simulink model "MA_simula_dsrac"  (R2012b)
settings: Solver=ode3  StartTime=0  StopTime=Tsim  FixedStep=1e-7  RelTol=1e-3
values from neighbouring files (symbols this model uses):
  D0 = 0.3    [MA_roda_sim.m]    (also in MF_roda_sim_disc.m; sim_padrao.mat = [0.344368016885 0.340474742468 0.337081858539 0.333995318743)
  dD = 0.01    [MA_roda_sim.m]
  dVin = 2    [MA_roda_sim.m]    (also in MF_roda_sim_disc.m)
  tdD = Tsim/3    (= 0.0333333333333)    [MA_roda_sim.m]
  tdVin = 2*Tsim/3    (= 0.0666666666667)    [MA_roda_sim.m]    (also in MF_roda_sim_disc.m = 0.2)
  Vin0 = 15.5    [MA_roda_sim.m]    (also in MF_roda_sim_disc.m)
undefined symbols (not defined in the file or in its folder): A_linear, B_mimo, C, tf_G_den, tf_G_num, tf_Gq_den, tf_Gq_num, xss
settings Model: CovModelRefEnable=off  Creator=jv_flores  LastModifiedBy=anton
settings DataIOCC: LimitDataPoints=off  SaveFormat=StructureWithTime
settings OptimizationCC: ExpressionDepthLimit=128
settings DebuggingCC: UnderspecifiedInitializationDetection=Simplified  MergeDetectMultiDrivingBlocksExec=error  SolverPrmCheckMsg=none  FrameProcessingCompatibilityMsg=error  StateNameClashWarn=none
settings HardwareCC: ProdBitPerPointer=64  ProdLargestAtomicFloat=Float  ProdIntDivRoundTo=Zero  ProdEndianess=LittleEndian  ProdHWDeviceType=Specified
settings ModelReferenceCC: PropagateSignalLabelsOutOfModel=on
settings CodeAppCC: CustomSymbolStrType=$N$R$M_T
settings GRTTargetCC: CodeReplacementLibrary=C89/C90 (ANSI)

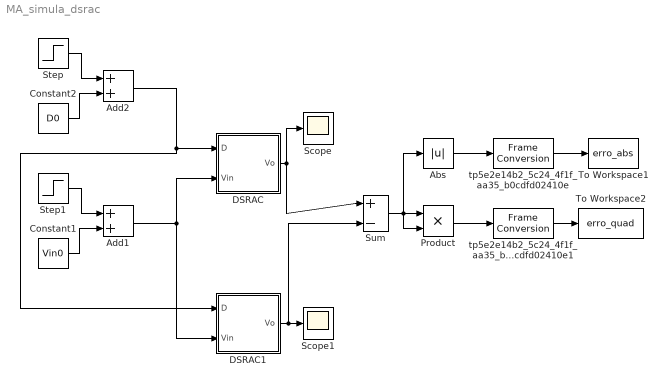
== system MA_simula_dsrac ==
  Abs : Abs
  Add1 : Sum
  Add2 : Sum
  Constant1 : Constant  Value=Vin0
  Constant2 : Constant  Value=D0
  DSRAC : Subsystem
  DSRAC1 : Subsystem
  Product : Product  RndMeth=Zero
  Scope : Scope
      settings: YMin=85.41748  YMax=114.83518
  Scope1 : Scope
      settings: YMin=85.41748  YMax=114.83518
  Step : Step  Time=tdD  After=dD  SampleTime=0
  Step1 : Step  Time=tdVin  After=dVin  SampleTime=0
  Sum : Sum  Inputs=|+-
  To Workspace1 : ToWorkspace  VariableName=erro_abs  SampleTime=-1
  To Workspace2 : ToWorkspace  VariableName=erro_quad  SampleTime=-1
  tp5e2e14b2_5c24_4f1f_aa35_b0cdfd02410e : FrameConversion  OutFrame=Sample-based
  tp5e2e14b2_5c24_4f1f_aa35_b0cdfd02410e1 : FrameConversion  OutFrame=Sample-based
  wires:
  DSRAC/1(Vo) -> Sum/1, Scope/1
  Step/1 -> Add2/1
  Constant2/1 -> Add2/2
  Add2/1 -> DSRAC1/1(D), DSRAC/1(D)
  Step1/1 -> Add1/1
  Constant1/1 -> Add1/2
  Add1/1 -> DSRAC/2(Vin), DSRAC1/2(Vin)
  DSRAC1/1(Vo) -> Sum/2, Scope1/1
  Sum/1 -> Abs/1, Product/2, Product/1
  tp5e2e14b2_5c24_4f1f_aa35_b0cdfd02410e/1 -> To Workspace1/1
  tp5e2e14b2_5c24_4f1f_aa35_b0cdfd02410e1/1 -> To Workspace2/1
  Product/1 -> tp5e2e14b2_5c24_4f1f_aa35_b0cdfd02410e1/1
  Abs/1 -> tp5e2e14b2_5c24_4f1f_aa35_b0cdfd02410e/1

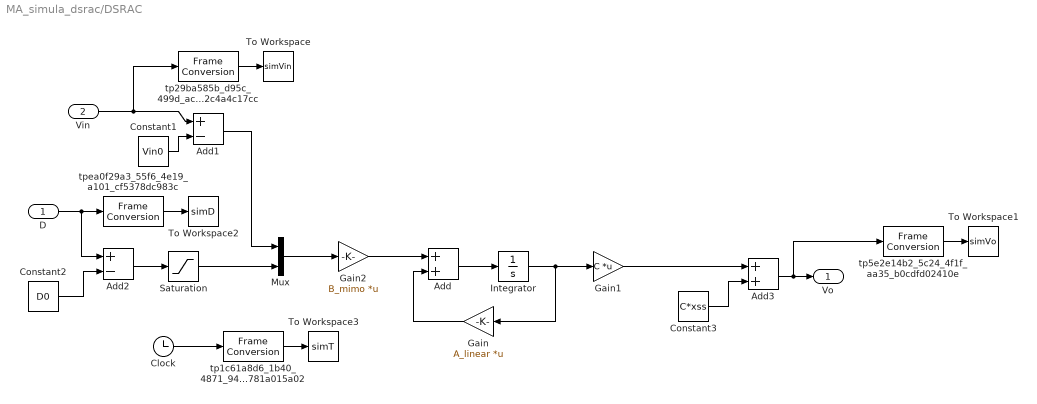
== system MA_simula_dsrac/DSRAC ==
  D : Inport
  Vin : Inport  Port=2
  Add : Sum
  Add1 : Sum  Inputs=+-
  Add2 : Sum  Inputs=+-
  Add3 : Sum
  Clock : Clock
  Constant1 : Constant  Value=Vin0
  Constant2 : Constant  Value=D0
  Constant3 : Constant  Value=C*xss
  Gain : Gain  Gain=A_linear  Multiplication=Matrix(K*u)
  Gain1 : Gain  Gain=C  Multiplication=Matrix(K*u)
  Gain2 : Gain  Gain=B_mimo  Multiplication=Matrix(K*u)
  Integrator : Integrator
  Mux : Mux  Inputs=2
  Saturation : Saturate  UpperLimit=1  LowerLimit=0
  To Workspace : ToWorkspace  VariableName=simVin  SampleTime=-1
  To Workspace1 : ToWorkspace  VariableName=simVo  SampleTime=-1
  To Workspace2 : ToWorkspace  VariableName=simD  SampleTime=-1
  To Workspace3 : ToWorkspace  VariableName=simT  SampleTime=-1
  tp1c61a8d6_1b40_4871_940a_a1781a015a02 : FrameConversion  OutFrame=Sample-based
  tp29ba585b_d95c_499d_aca0_992c4a4c17cc : FrameConversion  OutFrame=Sample-based
  tp5e2e14b2_5c24_4f1f_aa35_b0cdfd02410e : FrameConversion  OutFrame=Sample-based
  tpea0f29a3_55f6_4e19_a101_cf5378dc983c : FrameConversion  OutFrame=Sample-based
  Vo : Outport
  wires:
  Gain2/1 -> Add/1
  Add2/1 -> Saturation/1
  Constant2/1 -> Add2/2
  Integrator/1 -> Gain/1, Gain1/1
  Mux/1 -> Gain2/1
  Gain/1 -> Add/2
  Add/1 -> Integrator/1
  Add3/1 -> Vo/1, tp5e2e14b2_5c24_4f1f_aa35_b0cdfd02410e/1
  Gain1/1 -> Add3/1
  Constant3/1 -> Add3/2
  D/1 -> Add2/1, tpea0f29a3_55f6_4e19_a101_cf5378dc983c/1
  Saturation/1 -> Mux/2
  Vin/1 -> Add1/1, tp29ba585b_d95c_499d_aca0_992c4a4c17cc/1
  Constant1/1 -> Add1/2
  Add1/1 -> Mux/1
  tp29ba585b_d95c_499d_aca0_992c4a4c17cc/1 -> To Workspace/1
  tp5e2e14b2_5c24_4f1f_aa35_b0cdfd02410e/1 -> To Workspace1/1
  tpea0f29a3_55f6_4e19_a101_cf5378dc983c/1 -> To Workspace2/1
  Clock/1 -> tp1c61a8d6_1b40_4871_940a_a1781a015a02/1
  tp1c61a8d6_1b40_4871_940a_a1781a015a02/1 -> To Workspace3/1

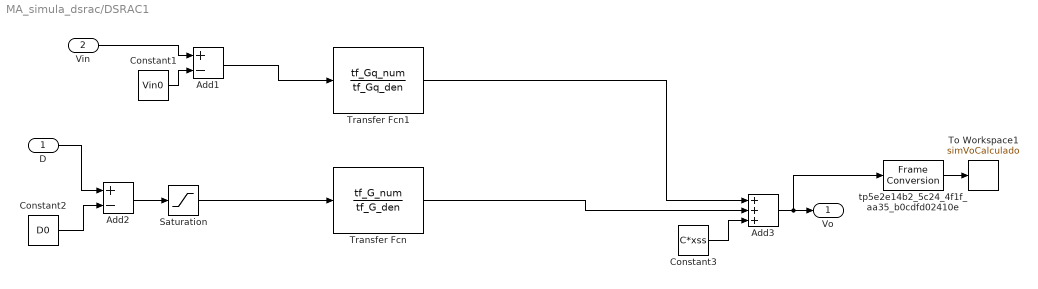
== system MA_simula_dsrac/DSRAC1 ==
  D : Inport
  Vin : Inport  Port=2
  Add1 : Sum  Inputs=+-
  Add2 : Sum  Inputs=+-
  Add3 : Sum  Inputs=+++
  Constant1 : Constant  Value=Vin0
  Constant2 : Constant  Value=D0
  Constant3 : Constant  Value=C*xss
  Saturation : Saturate  UpperLimit=1  LowerLimit=0
  To Workspace1 : ToWorkspace  VariableName=simVoCalculado  SampleTime=-1
  Transfer Fcn : TransferFcn  Numerator=tf_G_num  Denominator=tf_G_den
  Transfer Fcn1 : TransferFcn  Numerator=tf_Gq_num  Denominator=tf_Gq_den
  tp5e2e14b2_5c24_4f1f_aa35_b0cdfd02410e : FrameConversion  OutFrame=Sample-based
  Vo : Outport
  wires:
  Add2/1 -> Saturation/1
  Constant2/1 -> Add2/2
  Add3/1 -> Vo/1, tp5e2e14b2_5c24_4f1f_aa35_b0cdfd02410e/1
  Transfer Fcn1/1 -> Add3/1
  Constant3/1 -> Add3/3
  D/1 -> Add2/1
  Vin/1 -> Add1/1
  Constant1/1 -> Add1/2
  tp5e2e14b2_5c24_4f1f_aa35_b0cdfd02410e/1 -> To Workspace1/1
  Saturation/1 -> Transfer Fcn/1
  Add1/1 -> Transfer Fcn1/1
  Transfer Fcn/1 -> Add3/2
